simulink model "Control_System_Testbench_V1"  (R2018b)
settings: Solver=VariableStepAuto  StartTime=0.0  StopTime=100  RelTol=1e-3  EnableMultiTasking=on
undefined symbols (not defined in the file): A, B, C, Jw, K, R, reduction, sigbuilder_block
libraries: simulink x5
settings Model: Creator=univ4123  LastModifiedBy=univ4123
settings OptimizationCC: LifeSpan=inf
settings DebuggingCC: SFUnexpectedBacktrackingDiag=warning  SFNoUnconditionalDefaultTransitionDiag=warning
settings SFSimCC: SimUseLocalCustomCode=off
settings RTWCC: RTWUseLocalCustomCode=off
settings CodeAppCC: StateflowObjectComments=on
settings GRTTargetCC: TargetLangStandard=C89/C90 (ANSI)  GeneratePreprocessorConditionals=Disable all
settings ConfigComp: CovMetricSettings=dw  CovHtmlReporting=on  CovSaveCumulativeToWorkspaceVar=on  CovSaveSingleToWorkspaceVar=on  CovExternalEMLEnable=off

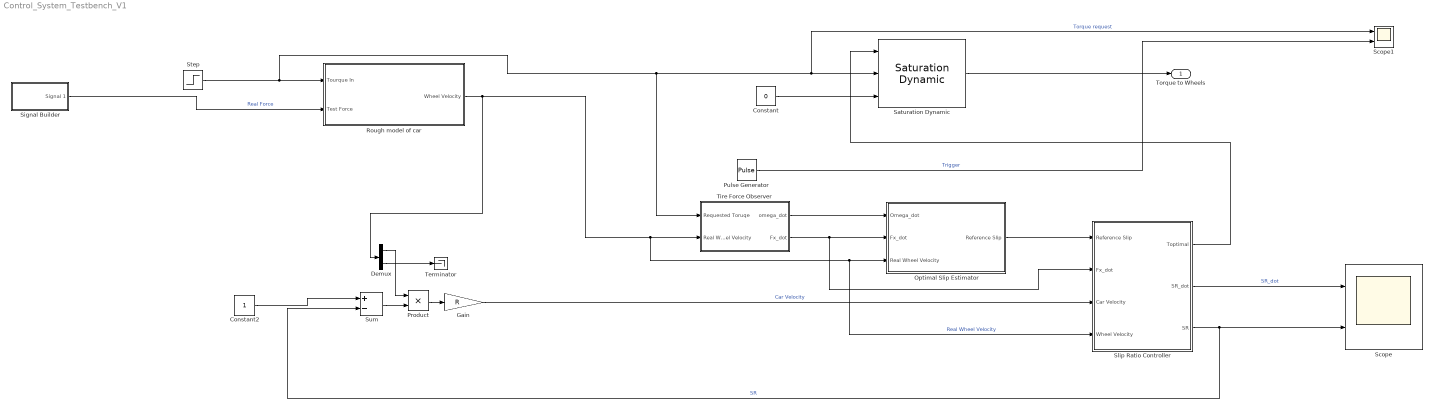
== system Control_System_Testbench_V1 ==
  Constant : Constant  Value=0
  Constant2 : Constant
  Demux : Demux  Outputs=2
  Gain : Gain  Gain=R
  Optimal Slip Estimator : Subsystem
  Product : Product
  Pulse Generator : DiscretePulseGenerator  PulseType=Time based  PulseWidth=5
  Rough model of car : Subsystem
  Saturation Dynamic : simulink/Discontinuities/Saturation Dynamic  OutMin=[]  OutMax=[]  OutDataTypeStr=Inherit: Same as second input  OutDataType=fixdt(1, 16)  OutScaling=2^-10  DoSatur=off
  Scope : Scope  NumInputPorts=2
  Scope1 : Scope  NumInputPorts=2
  Signal Builder : Subsystem  Tag=STV Subsys  LoadFcn=sigbuilder_block('load');  StartFcn=sigbuilder_block('start');  StopFcn=sigbuilder_block('stop');  ClipboardFcn=sigbuilder_block('clipboard');  mask(Sigbuilder block){tuvar=[0:10]}
      mask help: Simulink:masks:SigbuilderBlock_MD
      mask init:
      | if ~strcmp(get_param(bdroot(gcbh),'SimulationStatus'),'stopped') tuvar = sigbuilder_block('maskInit'); end
      settings: CopyFcn=sigbuilder_block('copy');  DeleteFcn=sigbuilder_block('delete');  ModelCloseFcn=sigbuilder_block('modelClose');  PreSaveFcn=sigbuilder_block('preSave');  PauseFcn=sigbuilder_block('pause');  ContinueFcn=sigbuilder_block('continue');  NameChangeFcn=sigbuilder_block('namechange');  OpenFcn=sigbuilder_block('open',[437.6 199.2 550.4 400 ]);  CloseFcn=sigbuilder_block('close');
      mask Display: plot(0, 0, 100, 100,[2, 2, 32, 32, 2], [68, 8, 8, 68, 68],[32, 2], [38, 38], [32, 19, 2],[53, 60, 44], [32, 17, 17, 2],[16, 16, 31, 31]);txt = getActiveGroup(gcbh);text(2, 100, txt,'verticalAlignment', 'top');
  Slip Ratio Controller : Subsystem
  Step : Step  After=5  SampleTime=0.001
  Sum : Sum  Inputs=+-
  Terminator : Terminator
  Tire Force Observer : Subsystem
  Torque to Wheels : Outport
  wires:
  Step/1 -> Tire Force Observer/1(Requested Toruqe), Scope1/1, Saturation Dynamic/2, Rough model of car/1(Tourque In)  "Torque request"
  Saturation Dynamic/1 -> Torque to Wheels/1
  Tire Force Observer/1(omega_dot) -> Optimal Slip Estimator/1(Omega_dot)
  Slip Ratio Controller/1(Toptimal) -> Saturation Dynamic/1
  Constant/1 -> Saturation Dynamic/3
  Tire Force Observer/2(Fx_dot) -> Slip Ratio Controller/2(Fx_dot), Optimal Slip Estimator/2(Fx_dot)
  Rough model of car/1(Wheel Velocity) -> Demux/1, Tire Force Observer/2(Real Wheel Velocity), Slip Ratio Controller/4(Wheel Velocity), Optimal Slip Estimator/3(Real Wheel Velocity)  "Real Wheel Velocity"
  Optimal Slip Estimator/1(Reference Slip) -> Slip Ratio Controller/1(Reference Slip)
  Gain/1 -> Slip Ratio Controller/3(Car Velocity)  "Car Velocity"
  Slip Ratio Controller/3(SR) -> Sum/2, Scope/2  "SR"
  Slip Ratio Controller/2(SR_dot) -> Scope/1  "SR_dot"
  Signal Builder/1(Signal 1) -> Rough model of car/2(Test Force)  "Real Force"
  Constant2/1 -> Sum/1
  Sum/1 -> Product/2
  Demux/1 -> Product/1
  Demux/2 -> Terminator/1
  Product/1 -> Gain/1
  Pulse Generator/1 -> Scope1/2  "Trigger"

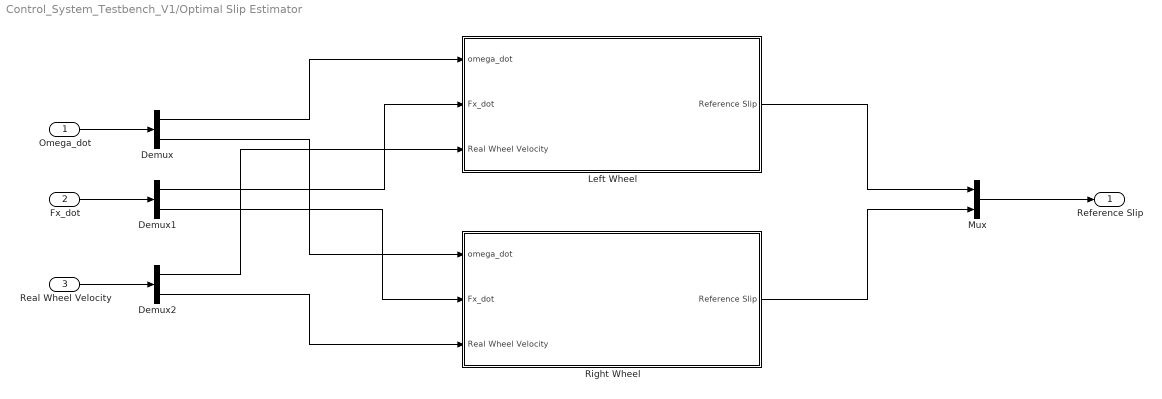
== system Control_System_Testbench_V1/Optimal Slip Estimator ==
  Omega_dot : Inport
  Fx_dot : Inport  Port=2
  Real Wheel Velocity : Inport  Port=3
  Demux : Demux  Outputs=2
  Demux1 : Demux  Outputs=2
  Demux2 : Demux  Outputs=2
  Left Wheel : Subsystem
  Mux : Mux  Inputs=2
  Right Wheel : Subsystem
  Reference Slip : Outport
  wires:
  Mux/1 -> Reference Slip/1
  Omega_dot/1 -> Demux/1
  Demux/1 -> Left Wheel/1(omega_dot)
  Demux/2 -> Right Wheel/1(omega_dot)
  Fx_dot/1 -> Demux1/1
  Real Wheel Velocity/1 -> Demux2/1
  Demux2/1 -> Left Wheel/3(Real Wheel Velocity)
  Demux2/2 -> Right Wheel/3(Real Wheel Velocity)
  Demux1/1 -> Left Wheel/2(Fx_dot)
  Demux1/2 -> Right Wheel/2(Fx_dot)
  Left Wheel/1(Reference Slip) -> Mux/1
  Right Wheel/1(Reference Slip) -> Mux/2

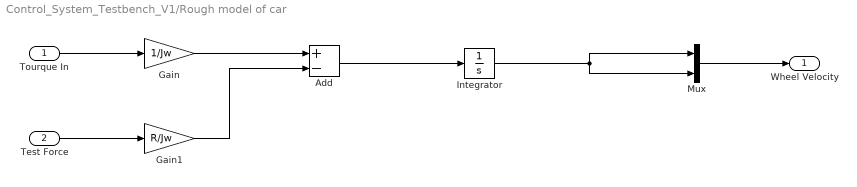
== system Control_System_Testbench_V1/Rough model of car ==
  Tourque In : Inport
  Test Force : Inport  Port=2
  Add : Sum  Inputs=+-
  Gain : Gain  Gain=1/Jw
  Gain1 : Gain  Gain=R/Jw
  Integrator : Integrator
  Mux : Mux  Inputs=2
  Wheel Velocity : Outport
  wires:
  Tourque In/1 -> Gain/1
  Gain/1 -> Add/1
  Test Force/1 -> Gain1/1
  Add/1 -> Integrator/1
  Gain1/1 -> Add/2
  Mux/1 -> Wheel Velocity/1
  Integrator/1 -> Mux/1, Mux/2

== system Control_System_Testbench_V1/Signal Builder ==
  Demux : Demux  Tag=STV Demux  Outputs=1
  FromWs : FromWorkspace  Tag=STV FromWs  VariableName=tuvar  SampleTime=0
      SigBuilderData=|
      | common.afterFinalStr = 'Extrapolate'
      | common.sampleTime = 0
      | dataSet.timeRange = [0 10]
      | dataSet.name = 'Group 1'
      | sbobj.Groups.Name = 'Group 1'
      | sbobj.Groups.Signals.Name = 'Signal 1'
      | sbobj.Groups.Signals.XData = [0 1 4 6 7 10]
      | sbobj.Groups.Signals.YData = [0 0 9.9 4.3 2.05 0]
  Signal 1 : Outport  Tag=STV Outport
  wires:
  Demux/1 -> Signal 1/1
  FromWs/1 -> Demux/1

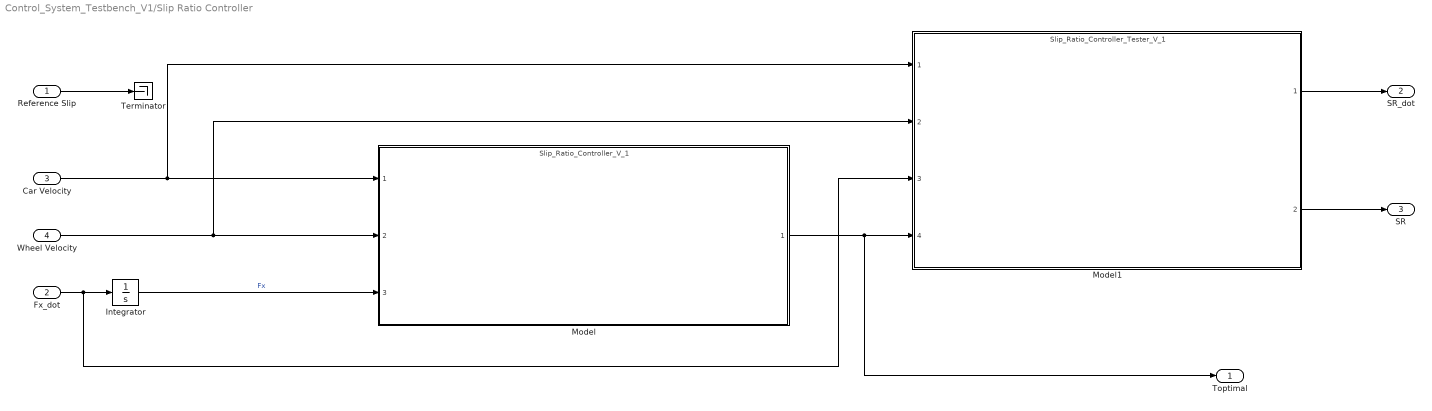
== system Control_System_Testbench_V1/Slip Ratio Controller ==
  Reference Slip : Inport
  Fx_dot : Inport  Port=2
  Car Velocity : Inport  Port=3
  Wheel Velocity : Inport  Port=4
  Integrator : Integrator
  Model : ModelReference  ModelNameDialog=Slip_Ratio_Controller_V_1.slx  SimulationMode=Normal  ModelReferenceVersion=1.9
  Model1 : ModelReference  ModelNameDialog=Slip_Ratio_Controller_Tester_V_1.slx  SimulationMode=Normal  ModelReferenceVersion=1.7
  Terminator : Terminator
  Toptimal : Outport
  SR_dot : Outport  Port=2
  SR : Outport  Port=3
  wires:
  Fx_dot/1 -> Model1/3, Integrator/1
  Integrator/1 -> Model/3  "Fx"
  Car Velocity/1 -> Model1/1, Model/1
  Wheel Velocity/1 -> Model1/2, Model/2
  Reference Slip/1 -> Terminator/1
  Model/1 -> Toptimal/1, Model1/4
  Model1/2 -> SR/1
  Model1/1 -> SR_dot/1

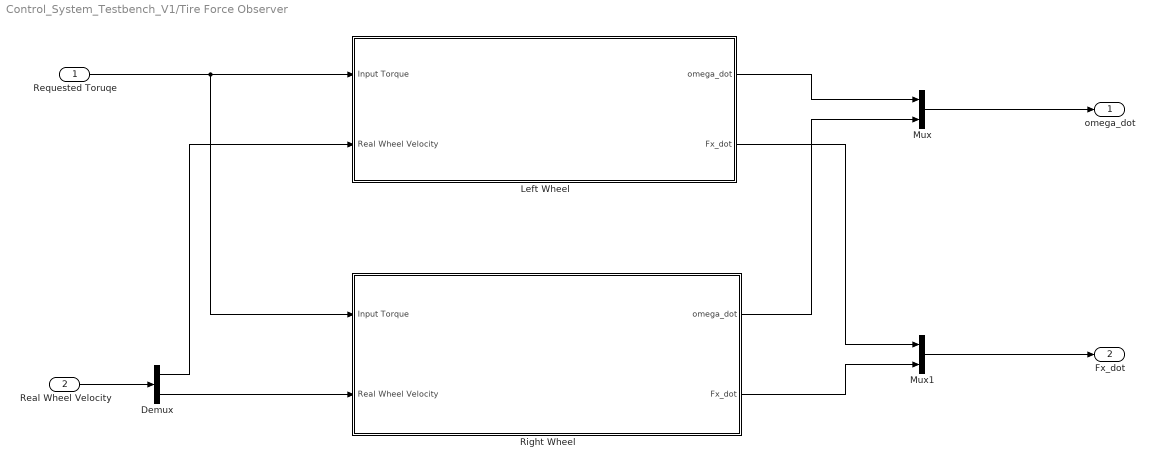
== system Control_System_Testbench_V1/Tire Force Observer ==
  Requested Toruqe : Inport
  Real Wheel Velocity : Inport  Port=2
  Demux : Demux  Outputs=2
  Left Wheel : Subsystem
  Mux : Mux  Inputs=2
  Mux1 : Mux  Inputs=2
  Right Wheel : Subsystem
  omega_dot : Outport
  Fx_dot : Outport  Port=2
  wires:
  Requested Toruqe/1 -> Right Wheel/1(Input Torque), Left Wheel/1(Input Torque)
  Real Wheel Velocity/1 -> Demux/1
  Demux/1 -> Left Wheel/2(Real Wheel Velocity)
  Demux/2 -> Right Wheel/2(Real Wheel Velocity)
  Right Wheel/1("omega_dot ") -> Mux/2
  Left Wheel/1("omega_dot ") -> Mux/1
  Left Wheel/2(Fx_dot) -> Mux1/1
  Right Wheel/2(Fx_dot) -> Mux1/2
  Mux/1 -> omega_dot/1
  Mux1/1 -> Fx_dot/1

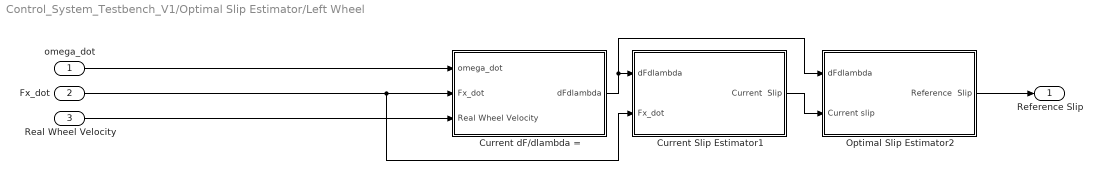
== system Control_System_Testbench_V1/Optimal Slip Estimator/Left Wheel ==
  omega_dot : Inport
  Fx_dot : Inport  Port=2
  Real Wheel Velocity : Inport  Port=3
  Current Slip Estimator1 : Subsystem
  Current dF/dlambda = : Subsystem
  Optimal Slip Estimator2 : Subsystem
  Reference Slip : Outport
  wires:
  Current dF/dlambda =/1(dFdlambda) -> Optimal Slip Estimator2/1("dFdlambda "), Current Slip Estimator1/1("dFdlambda ")
  Real Wheel Velocity/1 -> Current dF/dlambda =/3(Real Wheel Velocity)
  Fx_dot/1 -> Current Slip Estimator1/2(Fx_dot), Current dF/dlambda =/2(Fx_dot)
  omega_dot/1 -> Current dF/dlambda =/1(omega_dot)
  Current Slip Estimator1/1(" Current  Slip") -> Optimal Slip Estimator2/2("Current slip ")
  Optimal Slip Estimator2/1(" Reference  Slip") -> Reference Slip/1

== system Control_System_Testbench_V1/Optimal Slip Estimator/Right Wheel ==
  omega_dot : Inport
  Fx_dot : Inport  Port=2
  Real Wheel Velocity : Inport  Port=3
  Current Slip Estimator1 : Subsystem
  Current dF/dlambda = : Subsystem
  Optimal Slip Estimator2 : Subsystem
  Reference Slip : Outport
  wires:
  Current dF/dlambda =/1(dFdlambda) -> Optimal Slip Estimator2/1("dFdlambda "), Current Slip Estimator1/1("dFdlambda ")
  Real Wheel Velocity/1 -> Current dF/dlambda =/3(Real Wheel Velocity)
  Fx_dot/1 -> Current Slip Estimator1/2(Fx_dot), Current dF/dlambda =/2(Fx_dot)
  omega_dot/1 -> Current dF/dlambda =/1(omega_dot)
  Current Slip Estimator1/1(" Current  Slip") -> Optimal Slip Estimator2/2("Current slip ")
  Optimal Slip Estimator2/1(" Reference  Slip") -> Reference Slip/1

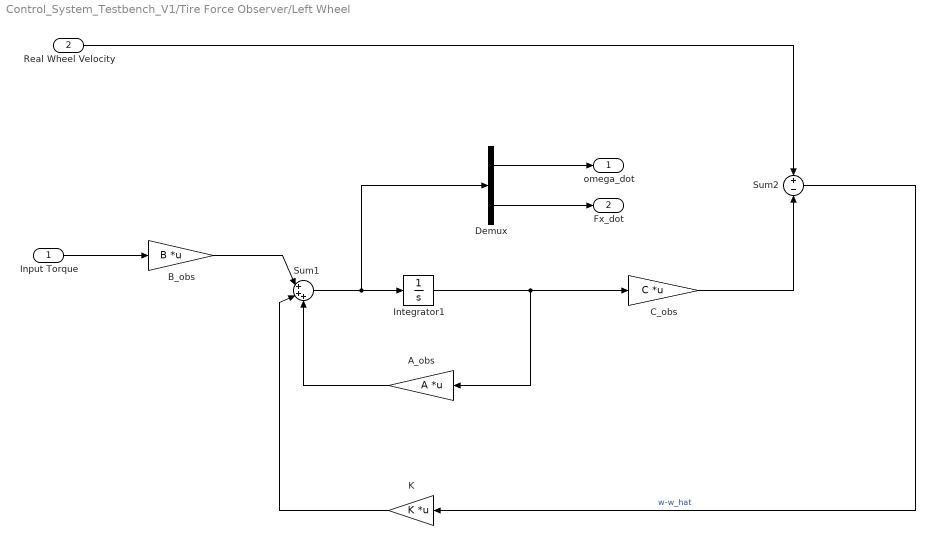
== system Control_System_Testbench_V1/Tire Force Observer/Left Wheel ==
  Input Torque : Inport
  Real Wheel Velocity : Inport  Port=2
  A_obs : Gain  Gain=A  Multiplication=Matrix(K*u) (u vector)
  B_obs : Gain  Gain=B  Multiplication=Matrix(K*u) (u vector)
  C_obs : Gain  Gain=C  Multiplication=Matrix(K*u) (u vector)
  Demux : Demux  Outputs=2
  Integrator1 : Integrator
  K : Gain  Gain=K  Multiplication=Matrix(K*u)
  Sum1 : Sum  Inputs=|+++
  Sum2 : Sum  Inputs=+|-
  "omega_dot " : Outport
  Fx_dot : Outport  Port=2
  wires:
  Demux/2 -> Fx_dot/1
  Input Torque/1 -> B_obs/1
  B_obs/1 -> Sum1/1
  Demux/1 -> "omega_dot "/1
  Sum1/1 -> Demux/1, Integrator1/1
  Integrator1/1 -> A_obs/1, C_obs/1
  A_obs/1 -> Sum1/3
  K/1 -> Sum1/2
  Sum2/1 -> K/1  "w-w_hat"
  Real Wheel Velocity/1 -> Sum2/1
  C_obs/1 -> Sum2/2

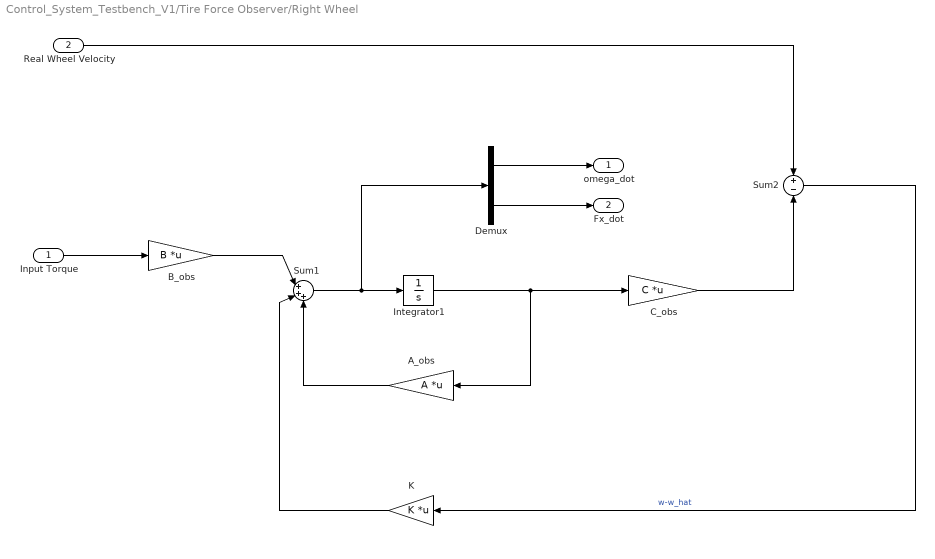
== system Control_System_Testbench_V1/Tire Force Observer/Right Wheel ==
  Input Torque : Inport
  Real Wheel Velocity : Inport  Port=2
  A_obs : Gain  Gain=A  Multiplication=Matrix(K*u) (u vector)
  B_obs : Gain  Gain=B  Multiplication=Matrix(K*u) (u vector)
  C_obs : Gain  Gain=C  Multiplication=Matrix(K*u) (u vector)
  Demux : Demux  Outputs=2
  Integrator1 : Integrator
  K : Gain  Gain=K  Multiplication=Matrix(K*u)
  Sum1 : Sum  Inputs=|+++
  Sum2 : Sum  Inputs=+|-
  "omega_dot " : Outport
  Fx_dot : Outport  Port=2
  wires:
  Demux/2 -> Fx_dot/1
  Input Torque/1 -> B_obs/1
  B_obs/1 -> Sum1/1
  Demux/1 -> "omega_dot "/1
  Sum1/1 -> Demux/1, Integrator1/1
  Integrator1/1 -> A_obs/1, C_obs/1
  A_obs/1 -> Sum1/3
  K/1 -> Sum1/2
  Sum2/1 -> K/1  "w-w_hat"
  Real Wheel Velocity/1 -> Sum2/1
  C_obs/1 -> Sum2/2

== system Control_System_Testbench_V1/Optimal Slip Estimator/Left Wheel/Current Slip Estimator1 ==
  "dFdlambda " : Inport
  Fx_dot : Inport  Port=2
  Integrator : Integrator
  Math Reciprocal : Math  Operator=reciprocal  SaturateOnIntegerOverflow=on
  Product : Product
  " Current  Slip" : Outport
  wires:
  "dFdlambda "/1 -> Math Reciprocal/1
  Fx_dot/1 -> Product/2
  Math Reciprocal/1 -> Product/1
  Product/1 -> Integrator/1
  Integrator/1 -> " Current  Slip"/1

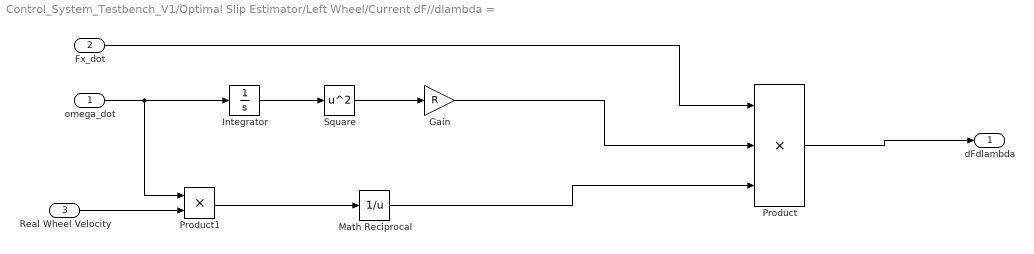
== system Control_System_Testbench_V1/Optimal Slip Estimator/Left Wheel/Current dF//dlambda = ==
  omega_dot : Inport
  Fx_dot : Inport  Port=2
  Real Wheel Velocity : Inport  Port=3
  Gain : Gain  Gain=R
  Integrator : Integrator
  Math Reciprocal : Math  Operator=reciprocal  SaturateOnIntegerOverflow=on
  Product : Product  Inputs=3
  Product1 : Product
  Square : Math  Operator=square  SaturateOnIntegerOverflow=on
  dFdlambda : Outport
  wires:
  omega_dot/1 -> Product1/1, Integrator/1
  Integrator/1 -> Square/1
  Square/1 -> Gain/1
  Fx_dot/1 -> Product/1
  Gain/1 -> Product/2
  Real Wheel Velocity/1 -> Product1/2
  Product1/1 -> Math Reciprocal/1
  Math Reciprocal/1 -> Product/3
  Product/1 -> dFdlambda/1

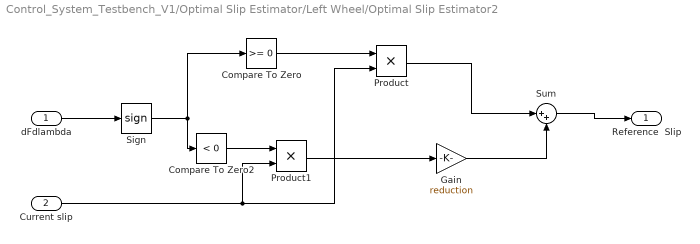
== system Control_System_Testbench_V1/Optimal Slip Estimator/Left Wheel/Optimal Slip Estimator2 ==
  "dFdlambda " : Inport
  "Current slip " : Inport  Port=2
  Compare To Zero : simulink/Logic and Bit Operations/Compare To Zero  relop=>=  OutDataTypeStr=boolean
  Compare To Zero2 : simulink/Logic and Bit Operations/Compare To Zero  relop=<  OutDataTypeStr=boolean
  Gain : Gain  Gain=reduction
  Product : Product
  Product1 : Product
  Sign : Signum
  Sum : Sum  Inputs=|++
  " Reference  Slip" : Outport
  wires:
  Sign/1 -> Compare To Zero2/1, Compare To Zero/1
  "dFdlambda "/1 -> Sign/1
  Compare To Zero2/1 -> Product1/1
  Gain/1 -> Sum/2
  Product/1 -> Sum/1
  Sum/1 -> " Reference  Slip"/1
  "Current slip "/1 -> Product1/2, Product/2
  Product1/1 -> Gain/1
  Compare To Zero/1 -> Product/1

== system Control_System_Testbench_V1/Optimal Slip Estimator/Right Wheel/Current Slip Estimator1 ==
  "dFdlambda " : Inport
  Fx_dot : Inport  Port=2
  Integrator : Integrator
  Math Reciprocal : Math  Operator=reciprocal  SaturateOnIntegerOverflow=on
  Product : Product
  " Current  Slip" : Outport
  wires:
  "dFdlambda "/1 -> Math Reciprocal/1
  Fx_dot/1 -> Product/2
  Math Reciprocal/1 -> Product/1
  Product/1 -> Integrator/1
  Integrator/1 -> " Current  Slip"/1

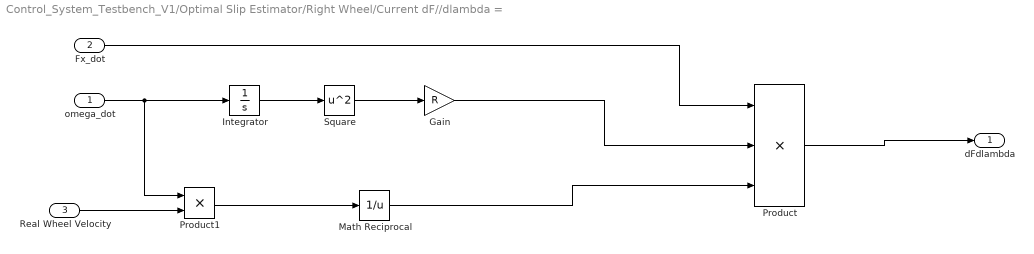
== system Control_System_Testbench_V1/Optimal Slip Estimator/Right Wheel/Current dF//dlambda = ==
  omega_dot : Inport
  Fx_dot : Inport  Port=2
  Real Wheel Velocity : Inport  Port=3
  Gain : Gain  Gain=R
  Integrator : Integrator
  Math Reciprocal : Math  Operator=reciprocal  SaturateOnIntegerOverflow=on
  Product : Product  Inputs=3
  Product1 : Product
  Square : Math  Operator=square  SaturateOnIntegerOverflow=on
  dFdlambda : Outport
  wires:
  omega_dot/1 -> Product1/1, Integrator/1
  Integrator/1 -> Square/1
  Square/1 -> Gain/1
  Fx_dot/1 -> Product/1
  Gain/1 -> Product/2
  Real Wheel Velocity/1 -> Product1/2
  Product1/1 -> Math Reciprocal/1
  Math Reciprocal/1 -> Product/3
  Product/1 -> dFdlambda/1

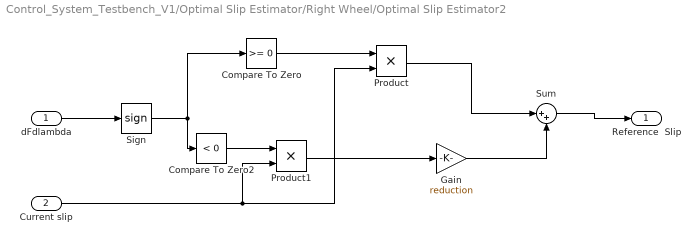
== system Control_System_Testbench_V1/Optimal Slip Estimator/Right Wheel/Optimal Slip Estimator2 ==
  "dFdlambda " : Inport
  "Current slip " : Inport  Port=2
  Compare To Zero : simulink/Logic and Bit Operations/Compare To Zero  relop=>=  OutDataTypeStr=boolean
  Compare To Zero2 : simulink/Logic and Bit Operations/Compare To Zero  relop=<  OutDataTypeStr=boolean
  Gain : Gain  Gain=reduction
  Product : Product
  Product1 : Product
  Sign : Signum
  Sum : Sum  Inputs=|++
  " Reference  Slip" : Outport
  wires:
  Sign/1 -> Compare To Zero2/1, Compare To Zero/1
  "dFdlambda "/1 -> Sign/1
  Compare To Zero2/1 -> Product1/1
  Gain/1 -> Sum/2
  Product/1 -> Sum/1
  Sum/1 -> " Reference  Slip"/1
  "Current slip "/1 -> Product1/2, Product/2
  Product1/1 -> Gain/1
  Compare To Zero/1 -> Product/1
